simulink model "ADIA"  (R2018b)
settings: Solver=FixedStepDiscrete  StartTime=0.0  StopTime=10.0  FixedStep=0.02  RelTol=1e-3
undefined symbols (not defined in the file or in its folder): ACC_State_Active, ACC_State_BrakeOnly, ACC_State_Suspended, ACC_State_WaitingRise, ADAS_AEBBrakingProg, ADAS_DeclControlReq, ADAS_DriveOff, ADAS_ESCHoldReq_NotHold, ADASDecType_ACC, ADASDecType_AEB, ADIA_ACC_Acceleration_OOR_DecCount_C, ADIA_ACC_Acceleration_OOR_Duration_C, ADIA_ACC_Acceleration_OOR_IncCount_C, ADIA_ACC_Acceleration_OOR_LLim_C, ADIA_ACC_Acceleration_OOR_ULim_C, ADIA_ACC_AccelTrqReq_MixedDia_ULim_C, ADIA_ACC_AccelTrqReq_ULim_C, ADIA_ACC_Deceleration_Mixed_ULim_C, ADIA_ACC_Deceleration_OOR_DecCount_C, ADIA_ACC_Deceleration_OOR_Duration_C, ADIA_ACC_Deceleration_OOR_IncCount_C, ADIA_ACC_Deceleration_OOR_LLim_C, ADIA_ACC_Deceleration_OOR_ULim_C, ADIA_ACC_DriveOff_Distance_C, ADIA_ACC_DriveOff_TimeLim_C, ADIA_ACC_ReqMixed_DecCount_C, ADIA_ACC_ReqMixed_Duration_C, ADIA_ACC_ReqMixed_IncCount_C, ADIA_AccPedalRaw_MaxLim_C, ADIA_AccPedalRaw_MinLim_C, ADIA_ADAS_HoldDecReq_Set_C, ADIA_ADAS_HoldRConfirm_TimeLim_C, ADIA_ADAS_HoldVehSpd_Lim_C, ADIA_AEB_VehSpdDec_LLim_C, ADIA_AEB_VehSpdDec_ULim_C, ADIA_ASWFault_OvrdEn_C, ADIA_ASWFault_OvrdValue_C, ADIA_BatteryOutOfRange_DecCount_C, ADIA_BatteryOutOfRange_Duration_C, ADIA_BatteryOutOfRange_IncCount_C, ADIA_BattVolt_MaxLim_C, ADIA_BattVolt_MinLim_C, ADIA_BCM3_33C_InvBrkLight_DecCount_C, ADIA_BCM3_33C_InvBrkLight_Duration_C, ADIA_BCM3_33C_InvBrkLight_IncCount_C, ADIA_BCM_BattVolt_OvrdEn_C, ADIA_BCM_BattVolt_OvrdVal_C, ADIA_BCM_BrakeLampStaus_OvrdEn_C, ADIA_BCM_BrakeLampStaus_OvrdVal_C, ADIA_BCM_CHMSLStaus_OvrdEn_C, ADIA_BCM_CHMSLStaus_OvrdVal_C, ADIA_BCM_LeftTurnSwSt_OvrdEn_C, ADIA_BCM_LeftTurnSwSt_OvrdVal_C, ADIA_BCM_RightTurnSwSt_OvrdEn_C, ADIA_BCM_RightTurnSwSt_OvrdVal_C, ADIA_BCM_TurnSwFailure_DecCount_C, ADIA_BCM_TurnSwFailure_Duration_C, ADIA_BCM_TurnSwFailure_IncCount_C, ADIA_BSWFault_Ignore_C, ADIA_BSWFault_OvrdEn_C ... (+281)
libraries: simulink x208
(part 3 of 10)

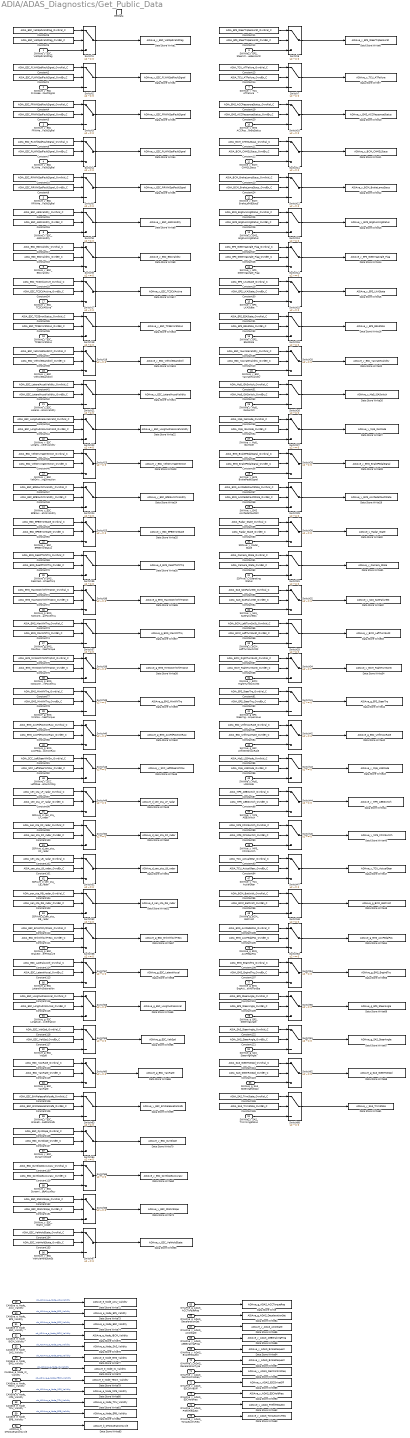
== system ADIA/ADAS_Diagnostics/Get_Public_Data ==
  SWINve_y_ESC_VehSpdValidFlag : Inport
  SWINve_y_ESC_FLWHeelSpdFaultSignal : Inport  Port=2
  SWINve_y_ESC_FRWHeelSpdFaultSignal : Inport  Port=3
  SWINve_y_ESC_RLWHeelSpdFaultSignal : Inport  Port=4
  SWINve_y_ESC_RRWHeelSpdFaultSignal : Inport  Port=5
  SWINve_y_EPS_SteerintTorqueSensorSt : Inport  Port=6
  SWINve_y_TCU_ATFailure : Inport  Port=7
  SWINve_y_ESC_ABSValidity : Inport  Port=8
  SWINve_y_ESC_ESCValidity : Inport  Port=9
  SWINve_y_EMS_ACCResponseStatus : Inport  Port=10
  SWINve_y_BCM_CHMSLStaus : Inport  Port=11
  SWINve_y_BCM_BrakeLampStaus : Inport  Port=12
  SWINve_y_EMS_EngRunningStatus : Inport  Port=13
  SWINve_y_EPS_SteeringAngle_Flag : Inport  Port=14
  SWINve_y_EPS_LKAState : Inport  Port=15
  SWINve_y_EPS_ESAState : Inport  Port=16
  SWINve_y_ESC_TCSCtlActive : Inport  Port=17
  SWINve_y_ESC_TCSErrorStatus : Inport  Port=18
  SWINve_y_ESC_VehicleStandstill : Inport  Port=19
  SWINve_y_ESC_YawrateValidity : Inport  Port=20
  SWINve_y_ESC_LateralAccelarationValidity : Inport  Port=21
  SWINve_y_ESC_LongitudinalAccelervalidity : Inport  Port=22
  SWINve_y_ESC_VehDrivingDirection : Inport  Port=23
  SWINve_y_ESC_EPBSwitchStaticsValidity : Inport  Port=24
  SWINve_y_ESC_EPBErrorStatus : Inport  Port=25
  SWINve_y_Mp5_ISASwitch : Inport  Port=26
  SWINve_y_Mp5_ISAMode : Inport  Port=27
  SWINve_y_EMS_BrakePedalSignal : Inport  Port=28
  SWINve_y_EMS_AccPedalFaultBit : Inport  Port=29
  SDFAve_y_Radar_State : Inport  Port=30
  SDFAve_y_OperatingStatus : Inport  Port=31
  SWINve_y_SAS_SASFailureSts : Inport  Port=32
  SWINve_y_BCM_LeftTurnSwitchSt : Inport  Port=33
  SWINve_y_BCM_RightTurnSwitchSt : Inport  Port=34
  SWINve_d_EMS_RealizedPowertrainWheelTorq : Inport  Port=35
  SWINve_g_EMS_NotControlableMaxPowertra : Inport  Port=36
  SWINve_g_EMS_MaxPowertrainWheelTorque : Inport  Port=37
  SWINve_g_EMS_NotControlableMinPowertra : Inport  Port=38
  SWINve_g_EMS_MinPowertrainWheelTorque : Inport  Port=39
  SWINve_g_EMS_AccPedalPositionRaw : Inport  Port=40
  SWINve_g_EPS_SteeringTorqueValue : Inport  Port=41
  SWINve_g_ESC_UnfilteredYawRate : Inport  Port=42  PortDimensions=1
  SWINve_y_Mp5_LSSMode : Inport  Port=43  OutDataTypeStr=uint8  PortDimensions=1
  SWINve_y_MP5_AEBSwitch : Inport  Port=44  OutDataTypeStr=uint8  PortDimensions=1
  SWINve_y_MP5_FCWSwitch : Inport  Port=45  OutDataTypeStr=uint8  PortDimensions=1
  SWINve_y_SCC_LeftSteeringWheelSwitchSig : Inport  Port=46  PortDimensions=1
  SWINve_y_TCU_ActialGear : Inport  Port=47  PortDimensions=1
  SWINve_g_BCM_BattVolt : Inport  Port=48  OutDataTypeStr=single  PortDimensions=1
  CANEve_e_Node_ACU_Validity : Inport  Port=49  PortDimensions=1
  CANEve_e_Node_EPS_Validity : Inport  Port=50  PortDimensions=1
  CANEve_e_Node_ESC_Validity : Inport  Port=51  PortDimensions=1
  CANEve_e_Node_IBCM_Validity : Inport  Port=52  PortDimensions=1
  CANEve_e_Node_SAS_Validity : Inport  Port=53  PortDimensions=1
  CANEve_e_Node_EMS_Validity : Inport  Port=54  PortDimensions=1
  CANEve_e_Node_IC_Validity : Inport  Port=55  PortDimensions=1
  CANEve_e_Node_TBOX_Validity : Inport  Port=56  PortDimensions=1
  CANEve_e_Node_MP5_Validity : Inport  Port=57  PortDimensions=1
  CANEve_e_Node_TCU_Validity : Inport  Port=58  PortDimensions=1
  CANEve_e_Node_EPB_Validity : Inport  Port=59  PortDimensions=1
  SDFAve_d_sen_sta_LF_radar : Inport  Port=60
  SDFAve_d_sen_sta_RF_radar : Inport  Port=61
  SDFAve_d_sen_sta_LB_radar : Inport  Port=62
  SDFAve_d_sen_sta_RB_radar : Inport  Port=63
  AFDMve_b_DTCOperationCycle : Inport  Port=64  OutDataTypeStr=T_BOOLEAN  PortDimensions=1
  OMAPve_g_ADAS_ACCTorqueReq : Inport  Port=65  OutDataTypeStr=T_M_Nm_Float32  PortDimensions=1
  OMAPve_g_ADAS_DecelerationSet : Inport  Port=66  OutDataTypeStr=T_M_Nm_Float32  PortDimensions=1
  OMAPve_y_ADAS_ACCState : Inport  Port=67  OutDataTypeStr=UInt8  PortDimensions=1
  OMAPve_y_ADAS_AEBBrakingProg : Inport  Port=68  OutDataTypeStr=UInt8  PortDimensions=1
  OMAPve_y_ADAS_BrakeRequest : Inport  Port=69  OutDataTypeStr=UInt8  PortDimensions=1
  OMAPve_y_ADAS_DecelerationType : Inport  Port=70  OutDataTypeStr=UInt8  PortDimensions=1
  OMAPve_y_ADAS_DeclControlReq : Inport  Port=71  OutDataTypeStr=UInt8  PortDimensions=1
  OMAPve_y_ADAS_ESCDriveOff : Inport  Port=72  OutDataTypeStr=UInt8  PortDimensions=1
  OMAPve_y_ADAS_ESCHoldReq : Inport  Port=73  OutDataTypeStr=UInt8  PortDimensions=1
  OMAPve_y_ADAS_PrefillRequest : Inport  Port=74  OutDataTypeStr=UInt8  PortDimensions=1
  OMAPve_y_ADAS_TorqueActivReq : Inport  Port=75  OutDataTypeStr=UInt8  PortDimensions=1
  SWINve_g_EMS_AccPedalPos : Inport  Port=76  OutDataTypeStr=single  PortDimensions=1
  SWINve_g_EMS_EngActualIndTorque : Inport  Port=77  OutDataTypeStr=single  PortDimensions=1
  SWINve_g_EPS_SteeringAngle : Inport  Port=78  OutDataTypeStr=single  PortDimensions=1
  SWINve_g_ESC_BrakeWheelCylinderPressure : Inport  Port=79  OutDataTypeStr=single  PortDimensions=1
  SWINve_g_ESC_LateralAccelaration : Inport  Port=80  OutDataTypeStr=single  PortDimensions=1
  SWINve_g_ESC_LongitudinalAcceleration : Inport  Port=81  OutDataTypeStr=single  PortDimensions=1
  SWINve_g_ESC_VeSpd : Inport  Port=82  OutDataTypeStr=single  PortDimensions=1
  SWINve_g_ESC_YawRate : Inport  Port=83  PortDimensions=1
  SWINve_g_SAS_SteeringAngle : Inport  Port=84  OutDataTypeStr=T_M_Nm_Float32  PortDimensions=1
  SWINve_g_SAS_SteeringRotSpd : Inport  Port=85  OutDataTypeStr=single  PortDimensions=1
  SWINve_y_ESC_BrakeReleasedFailsafe : Inport  Port=86  OutDataTypeStr=uint8  PortDimensions=1
  SWINve_y_ESC_DynamicSlope : Inport  Port=87  OutDataTypeStr=int8  PortDimensions=1
  SWINve_y_ESC_DynamicSlopeAccuracy : Inport  Port=88  OutDataTypeStr=uint8  PortDimensions=1
  SWINve_y_ESC_Static_slope : Inport  Port=89  OutDataTypeStr=int8  PortDimensions=1
  SWINve_y_ESC_VehicleHoldStatus : Inport  Port=90  OutDataTypeStr=uint8  PortDimensions=1
  SWINve_y_SAS_TrimmingStatus : Inport  Port=91  OutDataTypeStr=uint8  PortDimensions=1
  GetData : TriggerPort  TriggerType=function-call  VariantControl=(inherit)
  Constant1 : Constant  Value=ADIA_ESC_FLWhlSpdFaultSignal_OvrdEn_C
  Constant10 : Constant  Value=ADIA_ESC_RRWhlSpdFaultSignal_OvrdVal_C
  Constant100 : Constant  Value=ADIA_sen_sta_RF_radar_OvrdEn_C  OutDataTypeStr=T_BOOLEAN
  Constant101 : Constant  Value=ADIA_sen_sta_LB_radar_OvrdEn_C  OutDataTypeStr=T_BOOLEAN
  Constant102 : Constant  Value=ADIA_sen_sta_LB_radar_OvrdVal_C
  Constant103 : Constant  Value=ADIA_sen_sta_RB_radar_OvrdEn_C  OutDataTypeStr=T_BOOLEAN
  Constant104 : Constant  Value=ADIA_sen_sta_RB_radar_OvrdVal_C
  Constant105 : Constant  Value=ADIA_EMS_AccPedalPos_OvrdEn_C  OutDataTypeStr=T_BOOLEAN
  Constant106 : Constant  Value=ADIA_EMS_AccPedalPos_OvrdVal_C
  Constant107 : Constant  Value=ADIA_EMS_EngIndTrq_OvrdEn_C  OutDataTypeStr=T_BOOLEAN
  Constant108 : Constant  Value=ADIA_EMS_EngIndTrq_OvrdVal_C
  Constant109 : Constant  Value=ADIA_EPS_SteerAngle_OvrdEn_C  OutDataTypeStr=T_BOOLEAN
  Constant11 : Constant  Value=ADIA_EPS_SteerTrqSensorSt_OvrdVal_C
  Constant110 : Constant  Value=ADIA_EPS_SteerAngle_OvrdVal_C
  Constant111 : Constant  Value=ADIA_ESC_BrkWhlCylPress_OvrdEn_C  OutDataTypeStr=T_BOOLEAN
  Constant112 : Constant  Value=ADIA_ESC_BrkWhlCylPress_OvrdVal_C
  Constant113 : Constant  Value=ADIA_ESC_LateralAccel_OvrdEn_C  OutDataTypeStr=T_BOOLEAN
  Constant114 : Constant  Value=ADIA_ESC_LateralAccel_OvrdVal_C
  Constant115 : Constant  Value=ADIA_ESC_LongitudinalAccel_OvrdEn_C  OutDataTypeStr=T_BOOLEAN
  Constant116 : Constant  Value=ADIA_ESC_LongitudinalAccel_OvrdVal_C
  Constant117 : Constant  Value=ADIA_ESC_VehSpd_OvrdEn_C  OutDataTypeStr=T_BOOLEAN
  Constant118 : Constant  Value=ADIA_ESC_VehSpd_OvrdVal_C
  Constant119 : Constant  Value=ADIA_ESC_YawRate_OvrdEn_C  OutDataTypeStr=T_BOOLEAN
  Constant12 : Constant  Value=ADIA_EPS_SteerTrqSensorSt_OvrdEn_C
  Constant120 : Constant  Value=ADIA_ESC_YawRate_OvrdVal_C
  Constant121 : Constant  Value=ADIA_SAS_SteerAngle_OvrdEn_C  OutDataTypeStr=T_BOOLEAN
  Constant122 : Constant  Value=ADIA_SAS_SteerAngle_OvrdVal_C
  Constant123 : Constant  Value=ADIA_SAS_SteerRotSpd_OvrdEn_C  OutDataTypeStr=T_BOOLEAN
  Constant124 : Constant  Value=ADIA_SAS_SteerRotSpd_OvrdVal_C
  Constant125 : Constant  Value=ADIA_ESC_BrkReleaseFailsafe_OvrdEn_C  OutDataTypeStr=T_BOOLEAN
  Constant126 : Constant  Value=ADIA_ESC_BrkReleaseFailsafe_OvrdVal_C
  Constant127 : Constant  Value=ADIA_ESC_DynSlope_OvrdEn_C  OutDataTypeStr=T_BOOLEAN
  Constant128 : Constant  Value=ADIA_ESC_DynSlope_OvrdVal_C
  Constant129 : Constant  Value=ADIA_ESC_DynSlopeAccuracy_OvrdEn_C  OutDataTypeStr=T_BOOLEAN
  Constant13 : Constant  Value=ADIA_TCU_ATFailure_OvrdVal_C
  Constant130 : Constant  Value=ADIA_ESC_DynSlopeAccuracy_OvrdVal_C
  Constant131 : Constant  Value=ADIA_ESC_StaticSlope_OvrdEn_C  OutDataTypeStr=T_BOOLEAN
  Constant132 : Constant  Value=ADIA_ESC_StaticSlope_OvrdVal_C
  Constant133 : Constant  Value=ADIA_ESC_VehHoldState_OvrdEn_C  OutDataTypeStr=T_BOOLEAN
  Constant134 : Constant  Value=ADIA_ESC_VehHoldState_OvrdVal_C
  Constant135 : Constant  Value=ADIA_SAS_TrimState_OvrdEn_C  OutDataTypeStr=T_BOOLEAN
  Constant136 : Constant  Value=ADIA_SAS_TrimState_OvrdVal_C
  Constant14 : Constant  Value=ADIA_TCU_ATFailure_OvrdEn_C
  Constant15 : Constant  Value=ADIA_ESC_ABSValidity_OvrdVal_C
  Constant16 : Constant  Value=ADIA_ESC_ABSValidity_OvrdEn_C
  Constant17 : Constant  Value=ADIA_ESC_ESCValidity_OvrdVal_C
  Constant18 : Constant  Value=ADIA_ESC_ESCValidity_OvrdEn_C
  Constant19 : Constant  Value=ADIA_EMS_ACCResponseStatus_OvrdVal_C
  Constant2 : Constant  Value=ADIA_ESC_FLWhlSpdFaultSignal_OvrdVal_C
  Constant20 : Constant  Value=ADIA_EMS_ACCResponseStatus_OvrdEn_C
  Constant21 : Constant  Value=ADIA_BCM_CHMSLStaus_OvrdVal_C
  Constant22 : Constant  Value=ADIA_BCM_CHMSLStaus_OvrdEn_C
  Constant23 : Constant  Value=ADIA_BCM_BrakeLampStaus_OvrdVal_C
  Constant24 : Constant  Value=ADIA_BCM_BrakeLampStaus_OvrdEn_C
  Constant25 : Constant  Value=ADIA_EMS_EngRunningStatus_OvrdVal_C
  Constant26 : Constant  Value=ADIA_EMS_EngRunningStatus_OvrdEn_C
  Constant27 : Constant  Value=ADIA_EPS_SteeringAngle_Flag_OvrdVal_C
  Constant28 : Constant  Value=ADIA_EPS_SteeringAngle_Flag_OvrdEn_C
  Constant29 : Constant  Value=ADIA_EPS_LKAState_OvrdVal_C
  Constant3 : Constant  Value=ADIA_ESC_FRWhlSpdFaultSignal_OvrdEn_C
  Constant30 : Constant  Value=ADIA_EPS_LKAState_OvrdEn_C  OutDataTypeStr=T_BOOLEAN
  Constant31 : Constant  Value=ADIA_EPS_ESAState_OvrdVal_C
  Constant32 : Constant  Value=ADIA_EPS_ESAState_OvrdEn_C
  Constant33 : Constant  Value=ADIA_ESC_TCSCtlActive_OvrdVal_C
  Constant34 : Constant  Value=ADIA_ESC_TCSCtlActive_OvrdEn_C  OutDataTypeStr=T_BOOLEAN
  Constant35 : Constant  Value=ADIA_ESC_TCSErrorStatus_OvrdVal_C
  Constant36 : Constant  Value=ADIA_ESC_TCSErrorStatus_OvrdEn_C
  Constant37 : Constant  Value=ADIA_ESC_VehicleStandstill_OvrdVal_C
  Constant38 : Constant  Value=ADIA_ESC_VehicleStandstill_OvrdEn_C  OutDataTypeStr=T_BOOLEAN
  Constant39 : Constant  Value=ADIA_ESC_YawrateValidity_OvrdVal_C
  Constant4 : Constant  Value=ADIA_ESC_FRWhlSpdFaultSignal_OvrdVal_C
  Constant40 : Constant  Value=ADIA_ESC_YawrateValidity_OvrdEn_C  OutDataTypeStr=T_BOOLEAN
  Constant41 : Constant  Value=ADIA_ESC_LateralAccelValidity_OvrdVal_C
  Constant42 : Constant  Value=ADIA_ESC_LateralAccelValidity_OvrdEn_C  OutDataTypeStr=T_BOOLEAN
  Constant43 : Constant  Value=ADIA_ESC_LongitudinalAccelValid_OvrdVal_C
  Constant44 : Constant  Value=ADIA_ESC_LongitudinalAccelValid_OvrdEn_C  OutDataTypeStr=T_BOOLEAN
  Constant45 : Constant  Value=ADIA_ESC_VehDrivingDirection_OvrdVal_C
  Constant46 : Constant  Value=ADIA_ESC_VehDrivingDirection_OvrdEn_C  OutDataTypeStr=T_BOOLEAN
  Constant47 : Constant  Value=ADIA_ESC_EPBSwitchValidity_OvrdVal_C
  Constant48 : Constant  Value=ADIA_ESC_EPBSwitchValidity_OvrdEn_C  OutDataTypeStr=T_BOOLEAN
  Constant49 : Constant  Value=ADIA_ESC_EPBErrorState_OvrdVal_C
  Constant5 : Constant  Value=ADIA_ESC_VehSpdValidFlag_OvrdEn_C
  Constant50 : Constant  Value=ADIA_ESC_EPBErrorState_OvrdEn_C  OutDataTypeStr=T_BOOLEAN
  Constant51 : Constant  Value=ADIA_Mp5_ISASwitch_OvrdVal_C
  Constant52 : Constant  Value=ADIA_Mp5_ISASwitch_OvrdEn_C  OutDataTypeStr=T_BOOLEAN
  Constant53 : Constant  Value=ADIA_Mp5_ISAMode_OvrdVal_C
  Constant54 : Constant  Value=ADIA_Mp5_ISAMode_OvrdEn_C  OutDataTypeStr=T_BOOLEAN
  Constant55 : Constant  Value=ADIA_EMS_BrakePedalSignal_OvrdVal_C
  Constant56 : Constant  Value=ADIA_EMS_BrakePedalSignal_OvrdEn_C  OutDataTypeStr=T_BOOLEAN
  Constant57 : Constant  Value=ADIA_EMS_AccPedalFaultState_OvrdVal_C
  Constant58 : Constant  Value=ADIA_EMS_AccPedalFaultState_OvrdEn_C  OutDataTypeStr=T_BOOLEAN
  Constant59 : Constant  Value=ADIA_Radar_State_OvrdVal_C
  Constant6 : Constant  Value=ADIA_ESC_VehSpdValidFlag_OvrdVal_C
  Constant60 : Constant  Value=ADIA_Radar_State_OvrdEn_C  OutDataTypeStr=T_BOOLEAN
  Constant61 : Constant  Value=ADIA_Camera_State_OvrdVal_C
  Constant62 : Constant  Value=ADIA_Camera_State_OvrdEn_C  OutDataTypeStr=T_BOOLEAN
  Constant63 : Constant  Value=ADIA_SAS_SASFailureSt_OvrdVal_C
  Constant64 : Constant  Value=ADIA_SAS_SASFailureSt_OvrdEn_C  OutDataTypeStr=T_BOOLEAN
  Constant65 : Constant  Value=ADIA_BCM_LeftTurnSwSt_OvrdVal_C
  Constant66 : Constant  Value=ADIA_BCM_LeftTurnSwSt_OvrdEn_C  OutDataTypeStr=T_BOOLEAN
  Constant67 : Constant  Value=ADIA_BCM_RightTurnSwSt_OvrdVal_C
  Constant68 : Constant  Value=ADIA_BCM_RightTurnSwSt_OvrdEn_C  OutDataTypeStr=T_BOOLEAN
  Constant69 : Constant  Value=ADIA_EMS_RealPTWhlTrq_OvrdVal_C
  Constant7 : Constant  Value=ADIA_ESC_RLWhlSpdFaultSignal_OvrdEn_C
  Constant70 : Constant  Value=ADIA_EMS_RealPTWhlTrq_OvrdEn_C  OutDataTypeStr=T_BOOLEAN
  Constant71 : Constant  Value=ADIA_EMS_MaxNoCtrlWhlTrqOst_OvrdVal_C  OutDataTypeStr=Inherit: Inherit via back propagation
  Constant72 : Constant  Value=ADIA_EMS_MaxNoCtrlWhlTrqOst_OvrdEn_C  OutDataTypeStr=T_BOOLEAN
  Constant73 : Constant  Value=ADIA_EMS_MaxWhlTrq_OvrdVal_C
  Constant74 : Constant  Value=ADIA_EMS_MaxWhlTrq_OvrdEn_C  OutDataTypeStr=T_BOOLEAN
  Constant75 : Constant  Value=ADIA_EMS_MinNoCtrlWhlTrqOst_OvrdVal_C
  Constant76 : Constant  Value=ADIA_EMS_MinNoCtrlWhlTrqOst_OvrdEn_C  OutDataTypeStr=T_BOOLEAN
  Constant77 : Constant  Value=ADIA_EMS_MinWhlTrq_OvrdVal_C
  Constant78 : Constant  Value=ADIA_EMS_MinWhlTrq_OvrdEn_C  OutDataTypeStr=T_BOOLEAN
  Constant79 : Constant  Value=ADIA_EMS_AccPdPositionRaw_OvrdVal_C
  Constant8 : Constant  Value=ADIA_ESC_RLWhlSpdFaultSignal_OvrdVal_C
  Constant80 : Constant  Value=ADIA_EMS_AccPdPositionRaw_OvrdEn_C  OutDataTypeStr=T_BOOLEAN
  Constant81 : Constant  Value=ADIA_EPS_SteerTrq_OvrdVal_C
  Constant82 : Constant  Value=ADIA_EPS_SteerTrq_OvrdEn_C  OutDataTypeStr=T_BOOLEAN
  Constant83 : Constant  Value=ADIA_ESC_UnfltYawRate_OvrdVal_C
  Constant84 : Constant  Value=ADIA_ESC_UnfltYawRate_OvrdEn_C  OutDataTypeStr=T_BOOLEAN
  Constant85 : Constant  Value=ADIA_Mp5_LSSMode_OvrdVal_C
  Constant86 : Constant  Value=ADIA_Mp5_LSSMode_OvrdEn_C  OutDataTypeStr=T_BOOLEAN
  Constant87 : Constant  Value=ADIA_MP5_AEBSwitch_OvrdVal_C
  Constant88 : Constant  Value=ADIA_MP5_AEBSwitch_OvrdEn_C  OutDataTypeStr=T_BOOLEAN
  Constant89 : Constant  Value=ADIA_MP5_FCWSwitch_OvrdVal_C
  Constant9 : Constant  Value=ADIA_ESC_RRWhlSpdFaultSignal_OvrdEn_C
  Constant90 : Constant  Value=ADIA_MP5_FCWSwitch_OvrdEn_C  OutDataTypeStr=T_BOOLEAN
  Constant91 : Constant  Value=ADIA_SCC_LeftSteerWhlSw_OvrdVal_C
  Constant92 : Constant  Value=ADIA_SCC_LeftSteerWhlSw_OvrdEn_C  OutDataTypeStr=T_BOOLEAN
  Constant93 : Constant  Value=ADIA_TCU_ActualGear_OvrdVal_C
  Constant94 : Constant  Value=ADIA_TCU_ActualGear_OvrdEn_C  OutDataTypeStr=T_BOOLEAN
  Constant95 : Constant  Value=ADIA_BCM_BattVolt_OvrdVal_C
  Constant96 : Constant  Value=ADIA_BCM_BattVolt_OvrdEn_C
  Constant97 : Constant  Value=ADIA_sen_sta_LF_radar_OvrdVal_C
  Constant98 : Constant  Value=ADIA_sen_sta_LF_radar_OvrdEn_C  OutDataTypeStr=T_BOOLEAN
  Constant99 : Constant  Value=ADIA_sen_sta_RF_radar_OvrdVal_C
  Data Store Write : DataStoreWrite  DataStoreName=ADIAve_g_ADAS_ACCTorqueReq
  Data Store Write1 : DataStoreWrite  DataStoreName=ADIAve_y_ESC_VehSpdValidFlag
  Data Store Write10 : DataStoreWrite  DataStoreName=ADIAve_y_EMS_ACCResponseStatus
  Data Store Write11 : DataStoreWrite  DataStoreName=ADIAve_y_BCM_CHMSLStaus
  Data Store Write12 : DataStoreWrite  DataStoreName=ADIAve_y_BCM_BrakeLampStaus
  Data Store Write13 : DataStoreWrite  DataStoreName=ADIAve_y_EMS_EngRunningStatus
  Data Store Write14 : DataStoreWrite  DataStoreName=ADIAve_y_EPS_SteeringAngle_Flag
  Data Store Write15 : DataStoreWrite  DataStoreName=ADIAve_y_EPS_LKAState
  Data Store Write16 : DataStoreWrite  DataStoreName=ADIAve_y_EPS_ESAState
  Data Store Write17 : DataStoreWrite  DataStoreName=ADIAve_y_ESC_TCSCtlActive
  Data Store Write18 : DataStoreWrite  DataStoreName=ADIAve_y_ESC_TCSErrorStatus
  Data Store Write19 : DataStoreWrite  DataStoreName=ADIAve_y_ESC_VehicleStandstill
  Data Store Write2 : DataStoreWrite  DataStoreName=ADIAve_y_ESC_FLWhlSpdFaultSignal
  Data Store Write20 : DataStoreWrite  DataStoreName=ADIAve_y_ESC_YawrateValidity
  Data Store Write21 : DataStoreWrite  DataStoreName=ADIAve_y_ESC_LateralAccelValidity
  Data Store Write22 : DataStoreWrite  DataStoreName=ADIAve_y_ESC_LongitudinalAccelValidity
  Data Store Write23 : DataStoreWrite  DataStoreName=ADIAve_y_ESC_VehDrivingDirection
  Data Store Write24 : DataStoreWrite  DataStoreName=ADIAve_y_ESC_EPBSwitchValidity
  Data Store Write25 : DataStoreWrite  DataStoreName=ADIAve_y_ESC_EPBErrorState
  Data Store Write26 : DataStoreWrite  DataStoreName=ADIAve_y_Mp5_ISASwitch
  Data Store Write27 : DataStoreWrite  DataStoreName=ADIAve_y_Mp5_ISAMode
  Data Store Write28 : DataStoreWrite  DataStoreName=ADIAve_y_EMS_BrakePedalSignal
  Data Store Write29 : DataStoreWrite  DataStoreName=ADIAve_y_EMS_AccPedalFaultState
  Data Store Write3 : DataStoreWrite  DataStoreName=ADIAve_y_ESC_FRWhlSpdFaultSignal
  Data Store Write30 : DataStoreWrite  DataStoreName=ADIAve_y_Radar_State
  Data Store Write31 : DataStoreWrite  DataStoreName=ADIAve_y_Camera_State
  Data Store Write32 : DataStoreWrite  DataStoreName=ADIAve_y_SAS_SASFailureSt
  Data Store Write33 : DataStoreWrite  DataStoreName=ADIAve_y_BCM_LeftTurnSwSt
  Data Store Write34 : DataStoreWrite  DataStoreName=ADIAve_y_BCM_RightTurnSwSt
  Data Store Write35 : DataStoreWrite  DataStoreName=ADIAve_d_EMS_RealPTWhlTrq
  Data Store Write36 : DataStoreWrite  DataStoreName=ADIAve_g_EMS_MaxNoCtrlWhlTrqOst
  Data Store Write37 : DataStoreWrite  DataStoreName=ADIAve_g_EMS_MaxWhlTrq
  Data Store Write38 : DataStoreWrite  DataStoreName=ADIAve_g_EMS_MinNoCtrlWhlTrqOst
  Data Store Write39 : DataStoreWrite  DataStoreName=ADIAve_g_EMS_MinWhlTrq
  Data Store Write4 : DataStoreWrite  DataStoreName=ADIAve_y_ESC_RLWhlSpdFaultSignal
  Data Store Write40 : DataStoreWrite  DataStoreName=ADIAve_g_EMS_AccPdPositionRaw
  Data Store Write41 : DataStoreWrite  DataStoreName=ADIAve_g_EPS_SteerTrq
  Data Store Write42 : DataStoreWrite  DataStoreName=ADIAve_g_ESC_UnfltYawRate
  Data Store Write43 : DataStoreWrite  DataStoreName=ADIAve_y_Mp5_LSSMode
  Data Store Write44 : DataStoreWrite  DataStoreName=ADIAve_y_MP5_AEBSwitch
  Data Store Write45 : DataStoreWrite  DataStoreName=ADIAve_y_MP5_FCWSwitch
  Data Store Write46 : DataStoreWrite  DataStoreName=ADIAve_y_SCC_LeftSteerWhlSw
  Data Store Write47 : DataStoreWrite  DataStoreName=ADIAve_y_TCU_ActualGear
  Data Store Write48 : DataStoreWrite  DataStoreName=ADIAve_g_BCM_BattVolt
  Data Store Write49 : DataStoreWrite  DataStoreName=ADIAve_d_sen_sta_LF_radar
  Data Store Write5 : DataStoreWrite  DataStoreName=ADIAve_y_ESC_RRWhlSpdFaultSignal
  Data Store Write50 : DataStoreWrite  DataStoreName=ADIAve_d_sen_sta_RF_radar
  Data Store Write51 : DataStoreWrite  DataStoreName=ADIAve_d_sen_sta_LB_radar
  Data Store Write52 : DataStoreWrite  DataStoreName=ADIAve_d_sen_sta_RB_radar
  Data Store Write53 : DataStoreWrite  DataStoreName=ADIAve_y_ESC_VehHoldState
  Data Store Write54 : DataStoreWrite  DataStoreName=ADIAve_g_EMS_AccPedalPos
  Data Store Write55 : DataStoreWrite  DataStoreName=ADIAve_g_ESC_LongitudinalAccel
  Data Store Write56 : DataStoreWrite  DataStoreName=ADIAve_g_EMS_EngIndTrq
  Data Store Write57 : DataStoreWrite  DataStoreName=ADIAve_g_ESC_BrkWhlCylPress
  Data Store Write58 : DataStoreWrite  DataStoreName=ADIAve_g_ESC_LateralAccel
  Data Store Write59 : DataStoreWrite  DataStoreName=ADIAve_y_ESC_BrkReleaseFailsafe
  Data Store Write6 : DataStoreWrite  DataStoreName=ADIAve_y_EPS_SteerTrqSensorSt
  Data Store Write60 : DataStoreWrite  DataStoreName=ADIAve_y_ESC_DynSlopeAccuracy
  Data Store Write61 : DataStoreWrite  DataStoreName=ADIAve_y_SAS_TrimState
  Data Store Write62 : DataStoreWrite  DataStoreName=ADIAve_y_ADAS_PrefillRequest
  Data Store Write63 : DataStoreWrite  DataStoreName=ADIAve_y_ADAS_TorqueActivReq
  Data Store Write64 : DataStoreWrite  DataStoreName=ADIAve_y_ADAS_BrakeRequest
  Data Store Write65 : DataStoreWrite  DataStoreName=ADIAve_g_ESC_VehSpd
  Data Store Write66 : DataStoreWrite  DataStoreName=ADIAve_g_ESC_YawRate
  Data Store Write67 : DataStoreWrite  DataStoreName=ADIAve_g_SAS_SteerAngle
  Data Store Write68 : DataStoreWrite  DataStoreName=ADIAve_g_SAS_SteerRotSpd
  Data Store Write69 : DataStoreWrite  DataStoreName=ADIAve_g_EPS_SteerAngle
  Data Store Write7 : DataStoreWrite  DataStoreName=ADIAve_y_TCU_ATFailure
  Data Store Write70 : DataStoreWrite  DataStoreName=ADIAve_y_ESC_DynSlope
  Data Store Write71 : DataStoreWrite  DataStoreName=ADIAve_y_ESC_StaticSlope
  Data Store Write72 : DataStoreWrite  DataStoreName=ADIAve_e_Node_ACU_Validity
  Data Store Write73 : DataStoreWrite  DataStoreName=ADIAve_e_Node_EPS_Validity
  Data Store Write74 : DataStoreWrite  DataStoreName=ADIAve_e_Node_ESC_Validity
  Data Store Write75 : DataStoreWrite  DataStoreName=ADIAve_e_Node_IBCM_Validity
  Data Store Write76 : DataStoreWrite  DataStoreName=ADIAve_e_Node_SAS_Validity
  Data Store Write77 : DataStoreWrite  DataStoreName=ADIAve_e_Node_EMS_Validity
  Data Store Write78 : DataStoreWrite  DataStoreName=ADIAve_e_Node_IC_Validity
  Data Store Write79 : DataStoreWrite  DataStoreName=ADIAve_e_Node_TBOX_Validity
  Data Store Write8 : DataStoreWrite  DataStoreName=ADIAve_y_ESC_ABSValidity
  Data Store Write80 : DataStoreWrite  DataStoreName=ADIAve_e_Node_MP5_Validity
  Data Store Write81 : DataStoreWrite  DataStoreName=ADIAve_e_Node_TCU_Validity
  Data Store Write82 : DataStoreWrite  DataStoreName=ADIAve_e_Node_EPB_Validity
  Data Store Write83 : DataStoreWrite  DataStoreName=ADIAve_b_DTCOperationCycle
  Data Store Write84 : DataStoreWrite  DataStoreName=ADIAve_g_ADAS_DecelerationSet
  Data Store Write85 : DataStoreWrite  DataStoreName=ADIAve_y_ADAS_ACCState
  Data Store Write86 : DataStoreWrite  DataStoreName=ADIAve_y_ADAS_AEBBrakingProg
  Data Store Write87 : DataStoreWrite  DataStoreName=ADIAve_y_ADAS_BrakeRequest
  Data Store Write88 : DataStoreWrite  DataStoreName=ADIAve_y_ADAS_DeclControlReq
  Data Store Write89 : DataStoreWrite  DataStoreName=ADIAve_y_ADAS_ESCDriveOff
  Data Store Write9 : DataStoreWrite  DataStoreName=ADIAve_y_ESC_ESCValidity
  Data Store Write90 : DataStoreWrite  DataStoreName=ADIAve_y_ADAS_ESCHoldReq
  Switch{1..68} (68 alike) : Switch  Criteria=u2 ~= 0
  wires:
  Switch43/1 -> Data Store Write43/1
  Switch32/1 -> Data Store Write32/1
  Switch41/1 -> Data Store Write41/1
  Switch28/1 -> Data Store Write28/1
  Switch26/1 -> Data Store Write26/1
  Switch27/1 -> Data Store Write27/1
  Switch46/1 -> Data Store Write46/1
  Switch36/1 -> Data Store Write36/1
  Switch42/1 -> Data Store Write42/1
  Switch25/1 -> Data Store Write25/1
  Switch38/1 -> Data Store Write38/1
  Switch30/1 -> Data Store Write30/1
  Switch22/1 -> Data Store Write22/1
  Switch21/1 -> Data Store Write21/1
  Switch33/1 -> Data Store Write33/1
  Switch45/1 -> Data Store Write45/1
  Switch44/1 -> Data Store Write44/1
  Switch40/1 -> Data Store Write40/1
  CANEve_e_Node_ACU_Validity/1 -> Data Store Write72/1  "ob_ADIAve_e_Node_ACU_Validity"
  CANEve_e_Node_EPS_Validity/1 -> Data Store Write73/1  "ob_ADIAve_e_Node_EPS_Validity"
  CANEve_e_Node_ESC_Validity/1 -> Data Store Write74/1  "ob_ADIAve_e_Node_ESC_Validity"
  CANEve_e_Node_IBCM_Validity/1 -> Data Store Write75/1  "ob_ADIAve_e_Node_IBCM_Validity"
  CANEve_e_Node_SAS_Validity/1 -> Data Store Write76/1  "ob_ADIAve_e_Node_SAS_Validity"
  CANEve_e_Node_EMS_Validity/1 -> Data Store Write77/1  "ob_ADIAve_e_Node_EMS_Validity"
  CANEve_e_Node_IC_Validity/1 -> Data Store Write78/1  "ob_ADIAve_e_Node_IC_Validity"
  CANEve_e_Node_TBOX_Validity/1 -> Data Store Write79/1  "ob_ADIAve_e_Node_TBOX_Validity"
  CANEve_e_Node_MP5_Validity/1 -> Data Store Write80/1  "ob_ADIAve_e_Node_MP5_Validity"
  CANEve_e_Node_TCU_Validity/1 -> Data Store Write81/1  "ob_ADIAve_e_Node_TCU_Validity"
  CANEve_e_Node_EPB_Validity/1 -> Data Store Write82/1  "ob_ADIAve_e_Node_EPB_Validity"
  AFDMve_b_DTCOperationCycle/1 -> Data Store Write83/1
  Constant5/1 -> Switch1/2
  Constant6/1 -> Switch1/1
  SWINve_y_ESC_VehSpdValidFlag/1 -> Switch1/3
  Switch1/1 -> Data Store Write1/1
  Switch2/1 -> Data Store Write2/1
  Constant2/1 -> Switch2/1
  Constant1/1 -> Switch2/2
  SWINve_y_ESC_FLWHeelSpdFaultSignal/1 -> Switch2/3
  Constant3/1 -> Switch3/2
  Constant4/1 -> Switch3/1
  Switch3/1 -> Data Store Write3/1
  SWINve_y_ESC_FRWHeelSpdFaultSignal/1 -> Switch3/3
  Switch4/1 -> Data Store Write4/1
  Constant8/1 -> Switch4/1
  Constant7/1 -> Switch4/2
  SWINve_y_ESC_RLWHeelSpdFaultSignal/1 -> Switch4/3
  Constant9/1 -> Switch5/2
  Constant10/1 -> Switch5/1
  Switch5/1 -> Data Store Write5/1
  SWINve_y_ESC_RRWHeelSpdFaultSignal/1 -> Switch5/3
  Switch6/1 -> Data Store Write6/1
  Constant11/1 -> Switch6/1
  Constant12/1 -> Switch6/2
  SWINve_y_EPS_SteerintTorqueSensorSt/1 -> Switch6/3
  Switch7/1 -> Data Store Write7/1
  Constant13/1 -> Switch7/1
  Constant14/1 -> Switch7/2
  SWINve_y_TCU_ATFailure/1 -> Switch7/3
  Switch8/1 -> Data Store Write8/1
  Constant15/1 -> Switch8/1
  Constant16/1 -> Switch8/2
  SWINve_y_ESC_ABSValidity/1 -> Switch8/3
  Constant18/1 -> Switch9/2
  Constant17/1 -> Switch9/1
  Switch9/1 -> Data Store Write9/1
  SWINve_y_ESC_ESCValidity/1 -> Switch9/3
  Switch10/1 -> Data Store Write10/1
  Constant19/1 -> Switch10/1
  Constant20/1 -> Switch10/2
  SWINve_y_EMS_ACCResponseStatus/1 -> Switch10/3
  Switch11/1 -> Data Store Write11/1
  Constant21/1 -> Switch11/1
  Constant22/1 -> Switch11/2
  SWINve_y_BCM_CHMSLStaus/1 -> Switch11/3
  Switch12/1 -> Data Store Write12/1
  Constant23/1 -> Switch12/1
  Constant24/1 -> Switch12/2
  SWINve_y_BCM_BrakeLampStaus/1 -> Switch12/3
  Switch13/1 -> Data Store Write13/1
  Constant25/1 -> Switch13/1
  Constant26/1 -> Switch13/2
  SWINve_y_EMS_EngRunningStatus/1 -> Switch13/3
  Switch14/1 -> Data Store Write14/1
  Constant27/1 -> Switch14/1
  Constant28/1 -> Switch14/2
  SWINve_y_EPS_SteeringAngle_Flag/1 -> Switch14/3
  Constant30/1 -> Switch15/2
  Constant29/1 -> Switch15/1
  Switch15/1 -> Data Store Write15/1
  SWINve_y_EPS_LKAState/1 -> Switch15/3
  Switch16/1 -> Data Store Write16/1
  Constant31/1 -> Switch16/1
  Constant32/1 -> Switch16/2
  SWINve_y_EPS_ESAState/1 -> Switch16/3
  Switch17/1 -> Data Store Write17/1
  Constant33/1 -> Switch17/1
  Constant34/1 -> Switch17/2
  SWINve_y_ESC_TCSCtlActive/1 -> Switch17/3
  Constant36/1 -> Switch18/2
  Constant35/1 -> Switch18/1
  Switch18/1 -> Data Store Write18/1
  SWINve_y_ESC_TCSErrorStatus/1 -> Switch18/3
  Switch19/1 -> Data Store Write19/1
  Constant37/1 -> Switch19/1
  Constant38/1 -> Switch19/2
  SWINve_y_ESC_VehicleStandstill/1 -> Switch19/3
  Constant40/1 -> Switch20/2
  Constant39/1 -> Switch20/1
  Switch20/1 -> Data Store Write20/1
  SWINve_y_ESC_YawrateValidity/1 -> Switch20/3
  Constant42/1 -> Switch21/2
  Constant41/1 -> Switch21/1
  SWINve_y_ESC_LateralAccelarationValidity/1 -> Switch21/3
  Constant43/1 -> Switch22/1
  Constant44/1 -> Switch22/2
  SWINve_y_ESC_LongitudinalAccelervalidity/1 -> Switch22/3
  Constant46/1 -> Switch23/2
  Constant45/1 -> Switch23/1
  Switch23/1 -> Data Store Write23/1
  SWINve_y_ESC_VehDrivingDirection/1 -> Switch23/3
  Switch24/1 -> Data Store Write24/1
  Constant47/1 -> Switch24/1
  Constant48/1 -> Switch24/2
  SWINve_y_ESC_EPBSwitchStaticsValidity/1 -> Switch24/3
  Constant50/1 -> Switch25/2
  Constant49/1 -> Switch25/1
  SWINve_y_ESC_EPBErrorStatus/1 -> Switch25/3
  Constant51/1 -> Switch26/1
  Constant52/1 -> Switch26/2
  SWINve_y_Mp5_ISASwitch/1 -> Switch26/3
  Constant54/1 -> Switch27/2
  Constant53/1 -> Switch27/1
  SWINve_y_Mp5_ISAMode/1 -> Switch27/3
  Constant55/1 -> Switch28/1
  Constant56/1 -> Switch28/2
  SWINve_y_EMS_BrakePedalSignal/1 -> Switch28/3
  Constant58/1 -> Switch29/2
  Constant57/1 -> Switch29/1
  Switch29/1 -> Data Store Write29/1
  SWINve_y_EMS_AccPedalFaultBit/1 -> Switch29/3
  Constant59/1 -> Switch30/1
  Constant60/1 -> Switch30/2
  SDFAve_y_Radar_State/1 -> Switch30/3
  Constant62/1 -> Switch31/2
  Constant61/1 -> Switch31/1
  Switch31/1 -> Data Store Write31/1
  SDFAve_y_OperatingStatus/1 -> Switch31/3
  Constant63/1 -> Switch32/1
  Constant64/1 -> Switch32/2
  SWINve_y_SAS_SASFailureSts/1 -> Switch32/3
  Constant66/1 -> Switch33/2
  Constant65/1 -> Switch33/1
  SWINve_y_BCM_LeftTurnSwitchSt/1 -> Switch33/3
  Constant67/1 -> Switch34/1
  Constant68/1 -> Switch34/2
  Switch34/1 -> Data Store Write34/1
  SWINve_y_BCM_RightTurnSwitchSt/1 -> Switch34/3
  Constant69/1 -> Switch35/1
  Constant70/1 -> Switch35/2
  Switch35/1 -> Data Store Write35/1
  SWINve_d_EMS_RealizedPowertrainWheelTorq/1 -> Switch35/3
  Constant72/1 -> Switch36/2
  Constant71/1 -> Switch36/1
  SWINve_g_EMS_NotControlableMaxPowertra/1 -> Switch36/3
  Constant73/1 -> Switch37/1
  Constant74/1 -> Switch37/2
  Switch37/1 -> Data Store Write37/1
  SWINve_g_EMS_MaxPowertrainWheelTorque/1 -> Switch37/3
  Constant76/1 -> Switch38/2
  Constant75/1 -> Switch38/1
  SWINve_g_EMS_NotControlableMinPowertra/1 -> Switch38/3
  Constant77/1 -> Switch39/1
  Constant78/1 -> Switch39/2
  Switch39/1 -> Data Store Write39/1
  SWINve_g_EMS_MinPowertrainWheelTorque/1 -> Switch39/3
  Constant80/1 -> Switch40/2
  Constant79/1 -> Switch40/1
  SWINve_g_EMS_AccPedalPositionRaw/1 -> Switch40/3
  Constant82/1 -> Switch41/2
  Constant81/1 -> Switch41/1
  SWINve_g_EPS_SteeringTorqueValue/1 -> Switch41/3
  Constant83/1 -> Switch42/1
  Constant84/1 -> Switch42/2
  SWINve_g_ESC_UnfilteredYawRate/1 -> Switch42/3
  Constant85/1 -> Switch43/1
  Constant86/1 -> Switch43/2
  SWINve_y_Mp5_LSSMode/1 -> Switch43/3
  Constant88/1 -> Switch44/2
  Constant87/1 -> Switch44/1
  SWINve_y_MP5_AEBSwitch/1 -> Switch44/3
  Constant89/1 -> Switch45/1
  Constant90/1 -> Switch45/2
  SWINve_y_MP5_FCWSwitch/1 -> Switch45/3
  Constant92/1 -> Switch46/2
  Constant91/1 -> Switch46/1
  SWINve_y_SCC_LeftSteeringWheelSwitchSig/1 -> Switch46/3
  Constant94/1 -> Switch47/2
  Constant93/1 -> Switch47/1
  Switch47/1 -> Data Store Write47/1
  SWINve_y_TCU_ActialGear/1 -> Switch47/3
  Switch48/1 -> Data Store Write48/1
  Constant95/1 -> Switch48/1
  Constant96/1 -> Switch48/2
  SWINve_g_BCM_BattVolt/1 -> Switch48/3
  Constant97/1 -> Switch49/1
  Constant98/1 -> Switch49/2
  Switch49/1 -> Data Store Write49/1
  SDFAve_d_sen_sta_LF_radar/1 -> Switch49/3
  Switch50/1 -> Data Store Write50/1
  Constant100/1 -> Switch50/2
  Constant99/1 -> Switch50/1
  SDFAve_d_sen_sta_RF_radar/1 -> Switch50/3
  Constant102/1 -> Switch51/1
  Constant101/1 -> Switch51/2
  Switch51/1 -> Data Store Write51/1
  SDFAve_d_sen_sta_LB_radar/1 -> Switch51/3
  Switch52/1 -> Data Store Write52/1
  Constant103/1 -> Switch52/2
  Constant104/1 -> Switch52/1
  SDFAve_d_sen_sta_RB_radar/1 -> Switch52/3
  OMAPve_y_ADAS_DeclControlReq/1 -> Data Store Write88/1
  OMAPve_y_ADAS_AEBBrakingProg/1 -> Data Store Write86/1
  OMAPve_y_ADAS_DecelerationType/1 -> Data Store Write87/1
  OMAPve_y_ADAS_PrefillRequest/1 -> Data Store Write62/1
  OMAPve_y_ADAS_ESCHoldReq/1 -> Data Store Write90/1
  OMAPve_g_ADAS_DecelerationSet/1 -> Data Store Write84/1
  OMAPve_y_ADAS_ESCDriveOff/1 -> Data Store Write89/1
  OMAPve_y_ADAS_ACCState/1 -> Data Store Write85/1
  OMAPve_y_ADAS_BrakeRequest/1 -> Data Store Write64/1
  OMAPve_y_ADAS_TorqueActivReq/1 -> Data Store Write63/1
  OMAPve_g_ADAS_ACCTorqueReq/1 -> Data Store Write/1
  Constant106/1 -> Switch53/1
  Constant105/1 -> Switch53/2
  Switch53/1 -> Data Store Write54/1
  SWINve_g_EMS_AccPedalPos/1 -> Switch53/3
  Switch54/1 -> Data Store Write56/1
  Constant107/1 -> Switch54/2
  Constant108/1 -> Switch54/1
  SWINve_g_EMS_EngActualIndTorque/1 -> Switch54/3
  Constant110/1 -> Switch55/1
  Constant109/1 -> Switch55/2
  Switch55/1 -> Data Store Write69/1
  SWINve_g_EPS_SteeringAngle/1 -> Switch55/3
  Constant112/1 -> Switch56/1
  Constant111/1 -> Switch56/2
  Switch56/1 -> Data Store Write57/1
  SWINve_g_ESC_BrakeWheelCylinderPressure/1 -> Switch56/3
  Switch57/1 -> Data Store Write58/1
  Constant113/1 -> Switch57/2
  Constant114/1 -> Switch57/1
  SWINve_g_ESC_LateralAccelaration/1 -> Switch57/3
  Constant116/1 -> Switch58/1
  Constant115/1 -> Switch58/2
  Switch58/1 -> Data Store Write55/1
  SWINve_g_ESC_LongitudinalAcceleration/1 -> Switch58/3
  Switch59/1 -> Data Store Write65/1
  Constant117/1 -> Switch59/2
  Constant118/1 -> Switch59/1
  SWINve_g_ESC_VeSpd/1 -> Switch59/3
  Constant120/1 -> Switch60/1
  Constant119/1 -> Switch60/2
  Switch60/1 -> Data Store Write66/1
  SWINve_g_ESC_YawRate/1 -> Switch60/3
  Switch61/1 -> Data Store Write67/1
  Constant121/1 -> Switch61/2
  Constant122/1 -> Switch61/1
  SWINve_g_SAS_SteeringAngle/1 -> Switch61/3
  Constant124/1 -> Switch62/1
  Constant123/1 -> Switch62/2
  Switch62/1 -> Data Store Write68/1
  SWINve_g_SAS_SteeringRotSpd/1 -> Switch62/3
  Switch63/1 -> Data Store Write59/1
  Constant125/1 -> Switch63/2
  Constant126/1 -> Switch63/1
  SWINve_y_ESC_BrakeReleasedFailsafe/1 -> Switch63/3
  Constant128/1 -> Switch64/1
  Constant127/1 -> Switch64/2
  Switch64/1 -> Data Store Write70/1
  SWINve_y_ESC_DynamicSlope/1 -> Switch64/3
  Switch65/1 -> Data Store Write60/1
  Constant129/1 -> Switch65/2
  Constant130/1 -> Switch65/1
  SWINve_y_ESC_DynamicSlopeAccuracy/1 -> Switch65/3
  Constant132/1 -> Switch66/1
  Constant131/1 -> Switch66/2
  Switch66/1 -> Data Store Write71/1
  SWINve_y_ESC_Static_slope/1 -> Switch66/3
  Switch67/1 -> Data Store Write53/1
  Constant133/1 -> Switch67/2
  Constant134/1 -> Switch67/1
  SWINve_y_ESC_VehicleHoldStatus/1 -> Switch67/3
  Switch68/1 -> Data Store Write61/1
  Constant135/1 -> Switch68/2
  Constant136/1 -> Switch68/1
  SWINve_y_SAS_TrimmingStatus/1 -> Switch68/3

== system ADIA/ADAS_Diagnostics/Output_Processing ==
  Output : TriggerPort  TriggerType=function-call  VariantControl=(inherit)
  Bitwise Operator1 : simulink/Logic and Bit Operations/Bitwise Operator  logicop=NOT  UseBitMask=off  BitMask=bin2dec('11011001')  BitMaskRealWorld=Stored Integer
  Bitwise Operator2 : simulink/Logic and Bit Operations/Bitwise Operator  logicop=NOT  UseBitMask=off  BitMask=bin2dec('11011001')  BitMaskRealWorld=Stored Integer
  Bitwise Operator3 : simulink/Logic and Bit Operations/Bitwise Operator  logicop=AND  UseBitMask=off  NumInputPorts=2  BitMask=bin2dec('11011001')  BitMaskRealWorld=Stored Integer
  Bitwise Operator4 : simulink/Logic and Bit Operations/Bitwise Operator  logicop=AND  UseBitMask=off  NumInputPorts=2  BitMask=bin2dec('11011001')  BitMaskRealWorld=Stored Integer
  Bitwise Operator5 : simulink/Logic and Bit Operations/Bitwise Operator  logicop=NOT  UseBitMask=off  BitMask=bin2dec('11011001')  BitMaskRealWorld=Stored Integer
  Bitwise Operator6 : simulink/Logic and Bit Operations/Bitwise Operator  logicop=AND  UseBitMask=off  NumInputPorts=2  BitMask=bin2dec('11011001')  BitMaskRealWorld=Stored Integer
  Constant1 : Constant  Value=ADIA_FuncFault_Ignore_C  OutDataTypeStr=uint16
  Constant2 : Constant  Value=ADIA_BSWFault_Ignore_C
  Constant3 : Constant  Value=ADIA_FuncFault_OvrdValue_C  OutDataTypeStr=uint16
  Constant4 : Constant  Value=ADIA_FuncFault_OvrdEn_C  OutDataTypeStr=T_BOOLEAN
  Constant5 : Constant  Value=ADIA_ASWFault_OvrdEn_C
  Constant6 : Constant  Value=ADIA_ASWFault_OvrdValue_C
  Constant7 : Constant  Value=ADIA_BSWFault_OvrdEn_C
  Constant8 : Constant  Value=ADIA_BSWFault_OvrdValue_C
  Constant9 : Constant  Value=ADIA_BSWFault_Ignore_C
  Data Store Read : DataStoreRead  DataStoreName=ob_ADIAve_g_ASWFaultStatus_ini
  Data Store Read1 : DataStoreRead  DataStoreName=ob_ADIAve_d_FuncFaultStatus_ini
  Data Store Read2 : DataStoreRead  DataStoreName=ob_ADIAve_g_BSWFaultStatus_ini
  Data Type Conversion : DataTypeConversion
  Data Type Conversion1 : DataTypeConversion
  Data Type Conversion2 : DataTypeConversion
  Switch{1..6} (6 alike) : Switch  Criteria=u2 ~= 0
  ADIAve_g_ASWFaultStatus : Outport
  ADIAve_g_BSWFaultStatus : Outport  Port=2
  ADIAve_d_FuncFaultStatus : Outport  Port=3
  wires:
  Data Store Read/1 -> Bitwise Operator6/2, Switch6/3
  Constant9/1 -> Switch3/2, Bitwise Operator1/1
  Data Store Read2/1 -> Bitwise Operator4/2, Switch3/3
  Switch5/1 -> Switch4/3
  Constant4/1 -> Switch4/2
  Bitwise Operator4/1 -> Switch3/1
  Constant7/1 -> Switch2/2
  Bitwise Operator2/1 -> Bitwise Operator3/1
  Switch6/1 -> Switch1/3
  Constant6/1 -> Switch1/1
  Switch4/1 -> Data Type Conversion2/1  "ob_ADIAve_d_FuncFaultStatus"
  Bitwise Operator1/1 -> Bitwise Operator4/1
  Data Store Read1/1 -> Switch5/3, Bitwise Operator3/2
  Constant5/1 -> Switch1/2
  Constant1/1 -> Bitwise Operator2/1, Switch5/2
  Constant2/1 -> Bitwise Operator5/1, Switch6/2
  Bitwise Operator5/1 -> Bitwise Operator6/1
  Bitwise Operator6/1 -> Switch6/1
  Switch2/1 -> Data Type Conversion/1  "ob_ADIAve_g_BSWFaultStatus"
  Switch3/1 -> Switch2/3
  Constant8/1 -> Switch2/1
  Switch1/1 -> Data Type Conversion1/1  "ob_ADIAve_g_ASWFaultStatus"
  Constant3/1 -> Switch4/1
  Bitwise Operator3/1 -> Switch5/1
  Data Type Conversion1/1 -> ADIAve_g_ASWFaultStatus/1
  Data Type Conversion/1 -> ADIAve_g_BSWFaultStatus/1
  Data Type Conversion2/1 -> ADIAve_d_FuncFaultStatus/1

== system ADIA/ADAS_Diagnostics/Diagnostics_Processing/16Bits_Set1 ==
  Bit0 : Inport  OutDataTypeStr=boolean
  Bit1 : Inport  Port=2  OutDataTypeStr=boolean
  Bit2 : Inport  Port=3  OutDataTypeStr=boolean
  Bit3 : Inport  Port=4  OutDataTypeStr=boolean
  Bit4 : Inport  Port=5  OutDataTypeStr=boolean
  Bit5 : Inport  Port=6  OutDataTypeStr=boolean
  Bit6 : Inport  Port=7  OutDataTypeStr=boolean
  Bit7 : Inport  Port=8  OutDataTypeStr=boolean
  Bit8 : Inport  Port=9  OutDataTypeStr=boolean
  Bit9 : Inport  Port=10  OutDataTypeStr=boolean
  Bit10 : Inport  Port=11  OutDataTypeStr=boolean
  Bit11 : Inport  Port=12  OutDataTypeStr=boolean
  Bit12 : Inport  Port=13  OutDataTypeStr=boolean
  Bit13 : Inport  Port=14  OutDataTypeStr=boolean
  Bit14 : Inport  Port=15  OutDataTypeStr=boolean
  Bit15 : Inport  Port=16  OutDataTypeStr=boolean
  8Bits_Set : Subsystem
  8Bits_Set1 : Subsystem
  Add : Sum
  Data Type Conversion : DataTypeConversion  OutDataTypeStr=uint16
  Data Type Conversion1 : DataTypeConversion  OutDataTypeStr=uint16
  Shift Arithmetic : ArithShift  BitShiftNumber=8  BitShiftDirection=Left
  Index_16Bits : Outport  OutDataTypeStr=uint16
  wires:
  8Bits_Set1/1(Index_8Bits) -> Data Type Conversion1/1
  Shift Arithmetic/1 -> Add/2
  8Bits_Set/1(Index_8Bits) -> Data Type Conversion/1
  Add/1 -> Index_16Bits/1
  Data Type Conversion/1 -> Add/1
  Data Type Conversion1/1 -> Shift Arithmetic/1
  Bit0/1 -> 8Bits_Set/1(Bit0)
  Bit1/1 -> 8Bits_Set/2(Bit1)
  Bit2/1 -> 8Bits_Set/3(Bit2)
  Bit3/1 -> 8Bits_Set/4(Bit3)
  Bit4/1 -> 8Bits_Set/5(Bit4)
  Bit5/1 -> 8Bits_Set/6(Bit5)
  Bit6/1 -> 8Bits_Set/7(Bit6)
  Bit7/1 -> 8Bits_Set/8(Bit7)
  Bit8/1 -> 8Bits_Set1/1(Bit0)
  Bit9/1 -> 8Bits_Set1/2(Bit1)
  Bit10/1 -> 8Bits_Set1/3(Bit2)
  Bit11/1 -> 8Bits_Set1/4(Bit3)
  Bit12/1 -> 8Bits_Set1/5(Bit4)
  Bit13/1 -> 8Bits_Set1/6(Bit5)
  Bit14/1 -> 8Bits_Set1/7(Bit6)
  Bit15/1 -> 8Bits_Set1/8(Bit7)

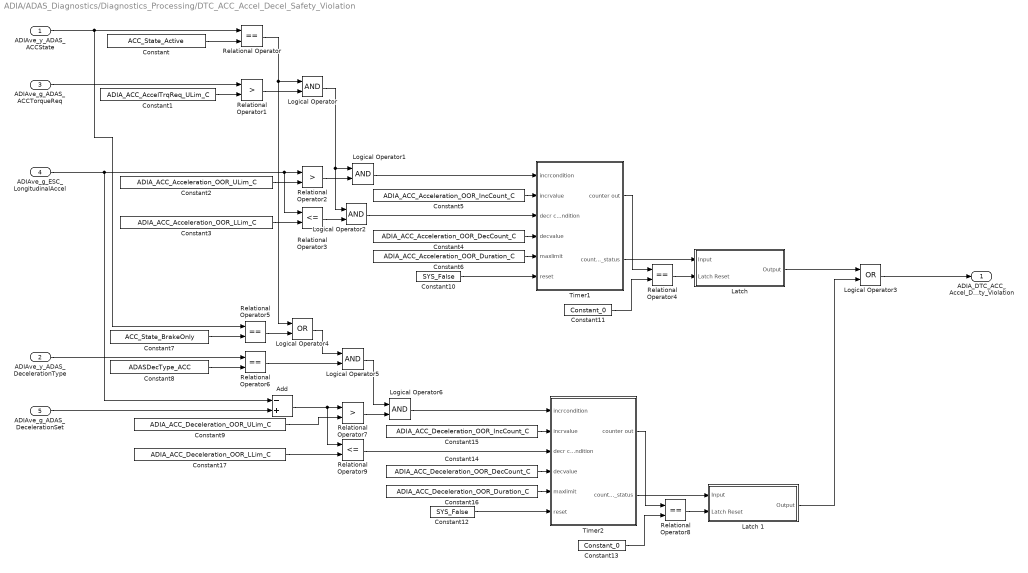
== system ADIA/ADAS_Diagnostics/Diagnostics_Processing/DTC_ACC_Accel_Decel_Safety_Violation ==
  ADIAve_y_ADAS_ACCState : Inport  OutDataTypeStr=UInt8  PortDimensions=1
  ADIAve_y_ADAS_DecelerationType : Inport  Port=2  OutDataTypeStr=UInt8  PortDimensions=1
  ADIAve_g_ADAS_ACCTorqueReq : Inport  Port=3  OutDataTypeStr=T_M_Nm_Float32  PortDimensions=1
  ADIAve_g_ESC_LongitudinalAccel : Inport  Port=4  OutDataTypeStr=single  PortDimensions=1
  ADIAve_g_ADAS_DecelerationSet : Inport  Port=5  OutDataTypeStr=T_M_Nm_Float32  PortDimensions=1
  Add : Sum  Inputs=-+
  Constant : Constant  Value=ACC_State_Active
  Constant1 : Constant  Value=ADIA_ACC_AccelTrqReq_ULim_C
  Constant10 : Constant  Value=SYS_False
  Constant11 : Constant  Value=Constant_0
  Constant12 : Constant  Value=SYS_False
  Constant13 : Constant  Value=Constant_0
  Constant14 : Constant  Value=ADIA_ACC_Deceleration_OOR_DecCount_C
  Constant15 : Constant  Value=ADIA_ACC_Deceleration_OOR_IncCount_C
  Constant16 : Constant  Value=ADIA_ACC_Deceleration_OOR_Duration_C
  Constant17 : Constant  Value=ADIA_ACC_Deceleration_OOR_LLim_C
  Constant2 : Constant  Value=ADIA_ACC_Acceleration_OOR_ULim_C
  Constant3 : Constant  Value=ADIA_ACC_Acceleration_OOR_LLim_C
  Constant4 : Constant  Value=ADIA_ACC_Acceleration_OOR_DecCount_C
  Constant5 : Constant  Value=ADIA_ACC_Acceleration_OOR_IncCount_C
  Constant6 : Constant  Value=ADIA_ACC_Acceleration_OOR_Duration_C
  Constant7 : Constant  Value=ACC_State_BrakeOnly
  Constant8 : Constant  Value=ADASDecType_ACC
  Constant9 : Constant  Value=ADIA_ACC_Deceleration_OOR_ULim_C
  "Latch " : Subsystem
  Latch 1 : Subsystem
  Logical Operator{,1..2,5..6} (5 alike) : Logic  AllPortsSameDT=off  OutDataTypeStr=boolean
  Logical Operator3 : Logic  Operator=OR  AllPortsSameDT=off  OutDataTypeStr=boolean
  Logical Operator4 : Logic  Operator=OR  AllPortsSameDT=off  OutDataTypeStr=boolean
  Relational Operator{,4..6,8} (5 alike) : RelationalOperator  Operator===  OutDataTypeStr=boolean  RndMeth=Simplest
  Relational Operator1 : RelationalOperator  Operator=>  OutDataTypeStr=boolean  RndMeth=Simplest
  Relational Operator2 : RelationalOperator  Operator=>  OutDataTypeStr=boolean  RndMeth=Simplest
  Relational Operator3 : RelationalOperator  Operator=<=  OutDataTypeStr=boolean  RndMeth=Simplest
  Relational Operator7 : RelationalOperator  Operator=>  OutDataTypeStr=boolean  RndMeth=Simplest
  Relational Operator9 : RelationalOperator  Operator=<=  OutDataTypeStr=boolean  RndMeth=Simplest
  Timer1 : Subsystem
  Timer2 : Subsystem
  ADIA_DTC_ACC_Accel_Decel_Safety_Violation : Outport
  wires:
  Constant/1 -> Relational Operator/2
  ADIAve_y_ADAS_ACCState/1 -> Relational Operator5/1, Relational Operator/1
  ADIAve_g_ADAS_ACCTorqueReq/1 -> Relational Operator1/1
  Constant1/1 -> Relational Operator1/2
  Relational Operator/1 -> Logical Operator4/1, Logical Operator/1
  Relational Operator1/1 -> Logical Operator/2
  Constant2/1 -> Relational Operator2/2
  Logical Operator/1 -> Logical Operator1/1, Logical Operator2/1
  Relational Operator2/1 -> Logical Operator1/2
  Logical Operator1/1 -> Timer1/1(incrcondition)
  Constant3/1 -> Relational Operator3/2
  ADIAve_g_ESC_LongitudinalAccel/1 -> Add/1, Relational Operator3/1, Relational Operator2/1
  Relational Operator3/1 -> Logical Operator2/2
  Logical Operator2/1 -> Timer1/3(decr condition)
  Constant10/1 -> Timer1/6(reset)
  Constant4/1 -> Timer1/4(decvalue)
  Constant5/1 -> Timer1/2(incrvalue)
  Constant11/1 -> Relational Operator4/2
  Relational Operator4/1 -> "Latch "/2(Latch Reset)
  Timer1/2(counter_status) -> "Latch "/1(Input)
  Timer1/1(counter out) -> Relational Operator4/1
  Constant6/1 -> Timer1/5(maxlimit)
  "Latch "/1(Output) -> Logical Operator3/1
  Constant7/1 -> Relational Operator5/2
  Relational Operator5/1 -> Logical Operator4/2
  Constant8/1 -> Relational Operator6/2
  Relational Operator6/1 -> Logical Operator5/2
  Logical Operator4/1 -> Logical Operator5/1
  ADIAve_y_ADAS_DecelerationType/1 -> Relational Operator6/1
  ADIAve_g_ADAS_DecelerationSet/1 -> Add/2
  Add/1 -> Relational Operator9/1, Relational Operator7/1
  Constant9/1 -> Relational Operator7/2
  Constant16/1 -> Timer2/5(maxlimit)
  Timer2/1(counter out) -> Relational Operator8/1
  Timer2/2(counter_status) -> Latch 1/1(Input)
  Relational Operator8/1 -> Latch 1/2(Latch Reset)
  Constant13/1 -> Relational Operator8/2
  Constant15/1 -> Timer2/2(incrvalue)
  Constant14/1 -> Timer2/4(decvalue)
  Constant12/1 -> Timer2/6(reset)
  Relational Operator9/1 -> Timer2/3(decr condition)
  Logical Operator6/1 -> Timer2/1(incrcondition)
  Logical Operator5/1 -> Logical Operator6/1
  Relational Operator7/1 -> Logical Operator6/2
  Constant17/1 -> Relational Operator9/2
  Logical Operator3/1 -> ADIA_DTC_ACC_Accel_Decel_Safety_Violation/1
  Latch 1/1(Output) -> Logical Operator3/2
